simulink model "sim_ex_wheelchair"  (R2016a)
settings: Solver=FixedStepAuto  StartTime=0.0  StopTime=3  FixedStep=0.01  RelTol=1e-3
model workspace: external: MAT-File (data not in the file)
settings Model: Creator=HYUNSOO  LastModifiedBy=Home
settings DataIOCC: LimitDataPoints=on  SaveFormat=Array
settings DebuggingCC: UnderspecifiedInitializationDetection=Classic  MergeDetectMultiDrivingBlocksExec=none  SolverPrmCheckMsg=warning  AllowSymbolicDim=off  StateNameClashWarn=warning
settings HardwareCC: ProdBitPerPointer=32  ProdLargestAtomicFloat=None  ProdIntDivRoundTo=Undefined  ProdEndianess=Unspecified  ProdWordSize=32  ProdHWDeviceType=32-bit Generic
settings ModelReferenceCC: PropagateSignalLabelsOutOfModel=off
settings ConfigComp: CovModelRefEnable=Off

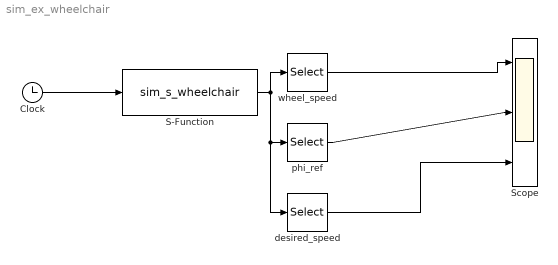
== system sim_ex_wheelchair ==
  Clock : Clock
  S-Function : S-Function  FunctionName=sim_s_wheelchair  Parameters=desire  SFunctionDeploymentMode=off  EnableBusSupport=off
  Scope : Scope  NumInputPorts=3
  desired_speed : Selector  InputPortWidth=6  IndexOptions=Index vector (dialog)  Indices=[4 5]  OutputSizes=1
  phi_ref : Selector  InputPortWidth=6  IndexOptions=Index vector (dialog)  Indices=[3 6]  OutputSizes=1
  wheel_speed : Selector  InputPortWidth=6  IndexOptions=Index vector (dialog)  Indices=[1 2]  OutputSizes=1
  wires:
  Clock/1 -> S-Function/1
  S-Function/1 -> desired_speed/1, phi_ref/1, wheel_speed/1
  wheel_speed/1 -> Scope/1
  phi_ref/1 -> Scope/2
  desired_speed/1 -> Scope/3
